simulink model "lab33"  (R2021b)
settings: Solver=VariableStepAuto  StartTime=0.0  StopTime=1.8  RelTol=1e-3
settings Model: Creator=asr77  LastModifiedBy=asr77

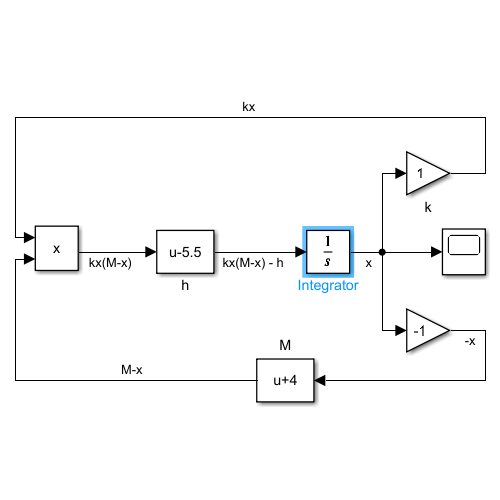
[thumbnail: Simulink's stored preview of the top-level diagram]
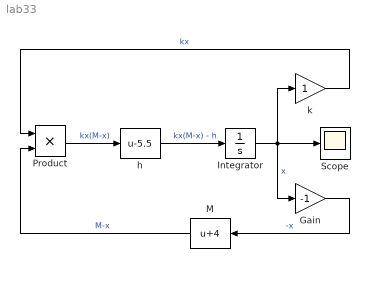
== system lab33 ==
  Gain : Gain  Gain=-1
  Integrator : Integrator  InitialCondition=3:0.5:5
  M : Bias  Bias=4
  Product : Product
  Scope : Scope
  h : Bias  Bias=-5.5
  k : Gain
  wires:
  Integrator/1 -> Scope/1, k/1, Gain/1  "x"
  Gain/1 -> M/1  "-x"
  M/1 -> Product/2  "M-x"
  k/1 -> Product/1  "kx"
  h/1 -> Integrator/1  "kx(M-x) - h"
  Product/1 -> h/1  "kx(M-x)"
